simulink model "HANcoder_E407_TTA_Group2"  (R2018b)
settings: Solver=FixedStepDiscrete  StartTime=0.0  StopTime=1  FixedStep=0.01  RelTol=1e-3
PreLoadFcn:
  | librarySetup
  | eval([bdroot,'_startup']) %Calling [modelName]_startup.m
values from neighbouring files (symbols this model uses):
  BackUp_Role = 4    [HANcoder_E407_TTA_Group2_startup.m]
  basic_cycle_duration_bc0 = TM_Reset_Board   + COMP_duration    (= 550)    [HANcoder_E407_TTA_Group2_startup.m]    (also in HANcoder_E407_TTA_Template_startup.m = 212)
  basic_cycle_duration_bc1 = TM_Reset_Var_bc1 + COMP_duration    (= 610)    [HANcoder_E407_TTA_Group2_startup.m]    (also in HANcoder_E407_TTA_Template_startup.m = 212)
  board1_online = Simulink.Parameter    [HANcoder_E407_TTA_Group2_startup.m]
  board2_online = Simulink.Parameter    [HANcoder_E407_TTA_Group2_startup.m]
  board3_online = Simulink.Parameter    [HANcoder_E407_TTA_Group2_startup.m]
  board4_online = Simulink.Parameter    [HANcoder_E407_TTA_Group2_startup.m]
  comm_delay_estimation1 = round(comm_delay_measured1*hardware_granularity/frequency_IRQ)    [HANcoder_E407_TTA_Group2_startup.m]    (also in HANcoder_E407_TTA_Template_startup.m)
  comm_delay_estimation2 = round(comm_delay_measured2*hardware_granularity/frequency_IRQ)    [HANcoder_E407_TTA_Group2_startup.m]    (also in HANcoder_E407_TTA_Template_startup.m)
  COMM_Period = 50    [HANcoder_E407_TTA_Group2_startup.m]    (also in HANcoder_E407_TTA_Template_startup.m = 40)
  COMM_Phase1 = Simulink.Parameter    [HANcoder_E407_TTA_Group2_startup.m]    (also in HANcoder_E407_TTA_Template_startup.m)
  COMM_Phase2 = Simulink.Parameter    [HANcoder_E407_TTA_Group2_startup.m]    (also in HANcoder_E407_TTA_Template_startup.m)
  COMM_Phase_init1 = Simulink.Parameter    [HANcoder_E407_TTA_Group2_startup.m]    (also in HANcoder_E407_TTA_Template_startup.m)
  COMM_Phase_init2 = Simulink.Parameter    [HANcoder_E407_TTA_Group2_startup.m]    (also in HANcoder_E407_TTA_Template_startup.m)
  COMP_duration = 20    [HANcoder_E407_TTA_Group2_startup.m]    (also in HANcoder_E407_TTA_Template_startup.m = 4)
  Controller1_Board = 1    [HANcoder_E407_TTA_Group2_startup.m]    (also in HANcoder_E407_TTA_Template_startup.m)
  Controller2_Board = 2    [HANcoder_E407_TTA_Group2_startup.m]    (also in HANcoder_E407_TTA_Template_startup.m)
  Controller3_Board = 3    [HANcoder_E407_TTA_Group2_startup.m]    (also in HANcoder_E407_TTA_Template_startup.m)
  Controller4_Board = 4    [HANcoder_E407_TTA_Group2_startup.m]
  delta_a_set = Simulink.Parameter    [HANcoder_E407_TTA_Group2_startup.m]
  delta_f_set = Simulink.Parameter    [HANcoder_E407_TTA_Group2_startup.m]
  delta_max = 1    [HANcoder_E407_TTA_Group2_startup.m]
  delta_min = -1    [HANcoder_E407_TTA_Group2_startup.m]
  delta_precision = 6    [HANcoder_E407_TTA_Group2_startup.m]
  e_width = 0.1    [HANcoder_E407_TTA_Group2_startup.m]
  ErrorLog_ID = 31    [HANcoder_E407_TTA_Group2_startup.m]
  frequency_IRQ = 100    [HANcoder_E407_TTA_Group2_startup.m]    (also in HANcoder_E407_TTA_Template_startup.m)
  HANtuneOverride = Simulink.Parameter    [HANcoder_E407_TTA_Group2_startup.m]    (also in HANcoder_E407_TTA_Template_startup.m)
  hardware_granularity = 1000000    [HANcoder_E407_TTA_Group2_startup.m]    (also in HANcoder_E407_TTA_Template_startup.m)
  I_a = 2.25    [HANcoder_E407_TTA_Group2_startup.m]
  I_f = 2.25    [HANcoder_E407_TTA_Group2_startup.m]
  idle_time_init = basic_cycle_duration_bc0 + basic_cycle_duration_bc1    (= 1160)    [HANcoder_E407_TTA_Group2_startup.m]    (also in HANcoder_E407_TTA_Template_startup.m = 424)
  Input_Gen_Board = 5    [HANcoder_E407_TTA_Group2_startup.m]
  LA_Clock_Gr = 1    [HANcoder_E407_TTA_Group2_startup.m]    (also in HANcoder_E407_TTA_Template_startup.m)
  LA_COMM_dly = 1    [HANcoder_E407_TTA_Group2_startup.m]    (also in HANcoder_E407_TTA_Template_startup.m)
  LA_COMM_Err = 1    [HANcoder_E407_TTA_Group2_startup.m]    (also in HANcoder_E407_TTA_Template_startup.m)
  LA_E_Desync = 1    [HANcoder_E407_TTA_Group2_startup.m]    (also in HANcoder_E407_TTA_Template_startup.m)
  LA_MEX_Flag = 1    [HANcoder_E407_TTA_Group2_startup.m]    (also in HANcoder_E407_TTA_Template_startup.m)
  LA_Task_Act = 1    [HANcoder_E407_TTA_Group2_startup.m]    (also in HANcoder_E407_TTA_Template_startup.m)
  m_v = 100.0    (= 100)    [HANcoder_E407_TTA_Group2_startup.m]
  Master_Role = 1    [HANcoder_E407_TTA_Group2_startup.m]    (also in HANcoder_E407_TTA_Template_startup.m)
  matrix_cycle_duration = basic_cycle_duration_bc0 + basic_cycle_duration_bc1    (= 1160)    [HANcoder_E407_TTA_Group2_startup.m]    (also in HANcoder_E407_TTA_Template_startup.m = 424)
  matrix_rows = 2    [HANcoder_E407_TTA_Group2_startup.m]    (also in HANcoder_E407_TTA_Template_startup.m)
  max_desync = 15    [HANcoder_E407_TTA_Group2_startup.m]    (also in HANcoder_E407_TTA_Template_startup.m)
  max_num_msgs_CAN1 = 2^Tx_bit_number-1    (= 7)    [HANcoder_E407_TTA_Group2_startup.m]    (also in HANcoder_E407_TTA_Template_startup.m)
  max_num_msgs_CAN2 = max_num_msgs_CAN1    (= 7)    [HANcoder_E407_TTA_Group2_startup.m]    (also in HANcoder_E407_TTA_Template_startup.m)
  min_desync = (-1)*max_desync    (= -15)    [HANcoder_E407_TTA_Group2_startup.m]    (also in HANcoder_E407_TTA_Template_startup.m)
  OutControl1_ID = 23    [HANcoder_E407_TTA_Group2_startup.m]    (also in HANcoder_E407_TTA_Template_startup.m)
  OutControl2_ID = 24    [HANcoder_E407_TTA_Group2_startup.m]    (also in HANcoder_E407_TTA_Template_startup.m)
  OutEmulator_ID = 25    [HANcoder_E407_TTA_Group2_startup.m]    (also in HANcoder_E407_TTA_Template_startup.m)
  R_al = 0.10    (= 0.1)    [HANcoder_E407_TTA_Group2_startup.m]
  R_ar = 0.10    (= 0.1)    [HANcoder_E407_TTA_Group2_startup.m]
  R_fl = 0.10    (= 0.1)    [HANcoder_E407_TTA_Group2_startup.m]
  R_fr = 0.10    (= 0.1)    [HANcoder_E407_TTA_Group2_startup.m]
  script_run = Simulink.Parameter    [HANcoder_E407_TTA_Group2_startup.m]    (also in HANcoder_E407_TTA_Template_startup.m)
  SensorValues_ID = 22    [HANcoder_E407_TTA_Group2_startup.m]    (also in HANcoder_E407_TTA_Template_startup.m)
  SetValues_ID = 21    [HANcoder_E407_TTA_Group2_startup.m]    (also in HANcoder_E407_TTA_Template_startup.m)
  Slave_Role = 3    [HANcoder_E407_TTA_Group2_startup.m]    (also in HANcoder_E407_TTA_Template_startup.m = 2)
  speed_k_d = Simulink.Parameter    [HANcoder_E407_TTA_Group2_startup.m]
  speed_k_i = Simulink.Parameter    [HANcoder_E407_TTA_Group2_startup.m]
  speed_k_p = Simulink.Parameter    [HANcoder_E407_TTA_Group2_startup.m]
  speed_max = 10    [HANcoder_E407_TTA_Group2_startup.m]
  speed_min = -10    [HANcoder_E407_TTA_Group2_startup.m]
  speed_precision = 3    [HANcoder_E407_TTA_Group2_startup.m]
  Sync_ID = 1    [HANcoder_E407_TTA_Group2_startup.m]    (also in HANcoder_E407_TTA_Template_startup.m)
  tau_max = 5    [HANcoder_E407_TTA_Group2_startup.m]
  tau_min = -5    [HANcoder_E407_TTA_Group2_startup.m]
  tau_range = abs(tau_max) + abs(tau_min)    [HANcoder_E407_TTA_Group2_startup.m]
  theta_max = (speed_max/R_fr)*matrix_cycle_duration*frequency_IRQ/hardware_granularity    (= 11.6)    [HANcoder_E407_TTA_Group2_startup.m]
  theta_min = (-1)*theta_max    (= -11.6)    [HANcoder_E407_TTA_Group2_startup.m]
  theta_precision = 7-(fix(log2(theta_max))+1)    [HANcoder_E407_TTA_Group2_startup.m]
  Tl_a = 0.6    [HANcoder_E407_TTA_Group2_startup.m]
  Tl_f = 0.6    [HANcoder_E407_TTA_Group2_startup.m]
  TM_bc0_1 = basic_cycle_start    (= 0)    [HANcoder_E407_TTA_Group2_startup.m]
  TM_bc0_10 = TM_bc0_9 + COMP_duration    (= 270)    [HANcoder_E407_TTA_Group2_startup.m]
  TM_bc0_11 = TM_bc0_10 + COMP_duration    (= 290)    [HANcoder_E407_TTA_Group2_startup.m]
  TM_bc0_12 = TM_bc0_11  + COMM_duration    (= 340)    [HANcoder_E407_TTA_Group2_startup.m]
  TM_bc0_13 = TM_bc0_12 + COMP_duration    (= 360)    [HANcoder_E407_TTA_Group2_startup.m]
  TM_bc0_14 = TM_bc0_13 + COMP_duration    (= 380)    [HANcoder_E407_TTA_Group2_startup.m]
  TM_bc0_15 = TM_bc0_14  + COMM_duration    (= 430)    [HANcoder_E407_TTA_Group2_startup.m]
  TM_bc0_16 = TM_bc0_15 + COMP_duration    (= 450)    [HANcoder_E407_TTA_Group2_startup.m]
  TM_bc0_17 = TM_bc0_16 + COMP_duration    (= 470)    [HANcoder_E407_TTA_Group2_startup.m]
  TM_bc0_18 = TM_bc0_17 + COMP_duration    (= 490)    [HANcoder_E407_TTA_Group2_startup.m]
  TM_bc0_2 = TM_bc0_1   + COMM_duration    (= 50)    [HANcoder_E407_TTA_Group2_startup.m]
  TM_bc0_3 = TM_bc0_2  + COMP_duration    (= 70)    [HANcoder_E407_TTA_Group2_startup.m]
  TM_bc0_3_2 = TM_bc0_3   + 2    (= 72)    [HANcoder_E407_TTA_Group2_startup.m]
  TM_bc0_4 = TM_bc0_3   + COMP_duration    (= 90)    [HANcoder_E407_TTA_Group2_startup.m]
  TM_bc0_4_2 = TM_bc0_4    + 2    (= 92)    [HANcoder_E407_TTA_Group2_startup.m]
  TM_bc0_5 = TM_bc0_4    + COMP_duration    (= 110)    [HANcoder_E407_TTA_Group2_startup.m]
  TM_bc0_6 = TM_bc0_5  + COMM_duration    (= 160)    [HANcoder_E407_TTA_Group2_startup.m]
  TM_bc0_7 = TM_bc0_6 + COMP_duration    (= 180)    [HANcoder_E407_TTA_Group2_startup.m]
  TM_bc0_8 = TM_bc0_7 + COMP_duration    (= 200)    [HANcoder_E407_TTA_Group2_startup.m]
  TM_bc0_9 = TM_bc0_8  + COMM_duration    (= 250)    [HANcoder_E407_TTA_Group2_startup.m]
  TM_bc0_9_2 = TM_bc0_9 + 2    (= 252)    [HANcoder_E407_TTA_Group2_startup.m]
  TM_bc1_18 = TM_Check_Output_Emulator + COMP_duration    (= 520)    [HANcoder_E407_TTA_Group2_startup.m]
  TM_bc1_19 = TM_bc1_18 + COMM_duration    (= 570)    [HANcoder_E407_TTA_Group2_startup.m]
  TM_bc1_19_2 = TM_bc1_19 + 2    (= 572)    [HANcoder_E407_TTA_Group2_startup.m]
  TM_Check_Output_Control1 = TM_COMM_Output_Control1 + COMP_duration    (= 340)    [HANcoder_E407_TTA_Group2_startup.m]
  TM_Check_Output_Control2 = TM_COMM_Output_Control2 + COMM_duration    (= 410)    [HANcoder_E407_TTA_Group2_startup.m]
  TM_Check_Output_Emulator = TM_COMM_Output_Emulator + COMM_duration    (= 500)    [HANcoder_E407_TTA_Group2_startup.m]
  TM_Check_Output_Emulator_2 = TM_Check_Output_Emulator + 2    (= 502)    [HANcoder_E407_TTA_Group2_startup.m]
  TM_Check_Sensor_Values = TM_COMM_Sensor_Values + COMM_duration    (= 210)    [HANcoder_E407_TTA_Group2_startup.m]
  TM_Check_Sensor_Values_2 = TM_Check_Sensor_Values + 2    (= 212)    [HANcoder_E407_TTA_Group2_startup.m]
  TM_Check_Set_Values = TM_COMM_Set_Values + COMM_duration    (= 140)    [HANcoder_E407_TTA_Group2_startup.m]
  TM_Check_Set_Values_2 = TM_Check_Set_Values + 2    (= 142)    [HANcoder_E407_TTA_Group2_startup.m]
  TM_COMM_Output_Control1 = TM_Velocity + COMM_duration    (= 320)    [HANcoder_E407_TTA_Group2_startup.m]
  TM_COMM_Output_Control2 = TM_Check_Output_Control1 + COMP_duration    (= 360)    [HANcoder_E407_TTA_Group2_startup.m]
  TM_COMM_Output_Emulator = TM_TMR + COMP_duration    (= 450)    [HANcoder_E407_TTA_Group2_startup.m]
  TM_COMM_Sensor_Values = TM_Check_Set_Values + COMP_duration    (= 160)    [HANcoder_E407_TTA_Group2_startup.m]
  TM_COMM_Set_Values = TM_bc0_3 + COMP_duration    (= 90)    [HANcoder_E407_TTA_Group2_startup.m]
  TM_COMM_Sync = basic_cycle_start    (= 0)    [HANcoder_E407_TTA_Group2_startup.m]    (also in HANcoder_E407_TTA_Template_startup.m)
  TM_Data_bc0 = TM_COMM_Sync    (= 0)    [HANcoder_E407_TTA_Group2_startup.m]    (also in HANcoder_E407_TTA_Template_startup.m)
  TM_Data_bc1 = TM_Data_bc0(1:4)    [HANcoder_E407_TTA_Group2_startup.m]    (also in HANcoder_E407_TTA_Template_startup.m)
  TM_Reset_Board = TM_Reset_Var   + COMP_duration    (= 530)    [HANcoder_E407_TTA_Group2_startup.m]    (also in HANcoder_E407_TTA_Template_startup.m = 208)
  TM_Reset_Var = TM_bc0_18  + COMP_duration    (= 510)    [HANcoder_E407_TTA_Group2_startup.m]    (also in HANcoder_E407_TTA_Template_startup.m = 204)
  TM_Reset_Var_bc1 = TM_bc1_19 + COMP_duration    (= 590)    [HANcoder_E407_TTA_Group2_startup.m]    (also in HANcoder_E407_TTA_Template_startup.m = 200)
  TM_Reset_Var_bc1_2 = TM_Reset_Var_bc1 + 2    (= 592)    [HANcoder_E407_TTA_Group2_startup.m]    (also in HANcoder_E407_TTA_Template_startup.m = 202)
  TM_Steer = TM_Check_Sensor_Values + COMP_duration    (= 230)    [HANcoder_E407_TTA_Group2_startup.m]
  TM_TMR = TM_Check_Output_Control2 + COMP_duration    (= 430)    [HANcoder_E407_TTA_Group2_startup.m]
  TM_TMR_2 = TM_TMR + 1    (= 431)    [HANcoder_E407_TTA_Group2_startup.m]
  ... (+19 more)
undefined symbols (not defined in the file or in its folder): A0, A1, A2, A3, A4, CON2, CON4, D10, D12, D13, D8, D9
libraries: hdlsllib x340, HANcoder_STM32_Target x28, simulink x5, simulink_extras x1
(part 27 of 36)

== system HANcoder_E407_TTA_Group2/HANcoder STM32 Target - E407-STM32 algorithm/TTA CAN System/TTA System/Matrix Cycle Manager/Vehicle Emulator Matrix Cycle/vehicle emulator basic cycle 1/COMM Task - Sensor_Values/Transmission subtasks/Check msg transmission CAN2 ==
  note: In the next tick, a message will be
      | sent through CAN2
  note: A message should be sent during
      | this tick through CAN2
  note: The TX buffers are updated one tick
      | before the message is sent
  Local Time : Inport
  Time Mark : Inport  Port=2
  Tx_ID : Inport  Port=3
  Value Domain Msg : Inport  Port=4
  Enable : EnablePort
  Constant : Constant  Value=COMM_Phase_init2
  Constant11 : Constant  Value=0
  Constant22 : Constant
  Constant24 : Constant  Value=COMM_Phase2
  Constant27 : Constant  Value=COMM_Phase2
  Constant8 : Constant  Value=0
  Equal4 : RelationalOperator  Operator===  OutDataTypeStr=boolean  RndMeth=Simplest
  Equal7 : RelationalOperator  Operator===  OutDataTypeStr=boolean  RndMeth=Simplest
  Minus : Sum  Inputs=++-
  Minus1 : Sum  Inputs=+-
  Minus2 : Sum
  Mod : Math  Operator=mod  SaturateOnIntegerOverflow=on
  Mod1 : Math  Operator=mod  SaturateOnIntegerOverflow=on
  TX buffer update CAN2 : Subsystem  Priority=20
  Send CAN2 : Outport  OutputWhenDisabled=reset  InitialOutput=0
  wires:
  Constant8/1 -> Equal4/2
  Equal7/1 -> Send CAN2/1
  Constant11/1 -> Equal7/2
  Minus1/1 -> Mod1/1
  Mod/1 -> Equal4/1
  Constant24/1 -> Mod/2
  Value Domain Msg/1 -> TX buffer update CAN2/2(Msg_Value_Data)
  Minus/1 -> Mod/1
  Constant27/1 -> Mod1/2
  Mod1/1 -> Equal7/1
  Tx_ID/1 -> TX buffer update CAN2/1(Tx_ID)
  Local Time/1 -> Minus/1, Minus1/1
  Constant22/1 -> Minus/2
  Equal4/1 -> TX buffer update CAN2/Enable
  Constant/1 -> Minus2/2
  Time Mark/1 -> Minus2/1
  Minus2/1 -> Minus1/2, Minus/3

== system HANcoder_E407_TTA_Group2/HANcoder STM32 Target - E407-STM32 algorithm/TTA CAN System/TTA System/Matrix Cycle Manager/Vehicle Emulator Matrix Cycle/vehicle emulator basic cycle 1/COMM Task - Sensor_Values/Transmission subtasks/Msg_Value_Data_Encoded ==
  note: Value domain message encoding
      | <Warning!> The first buffer (from the top) is not used in transmission!
  Enable : EnablePort
  Bus Creator : BusCreator  Inputs=8  OutDataTypeStr=Bus: msg_buffer_type
  Constant : Constant  Value=0  OutDataTypeStr=uint8
  Constant{1,7,10,13} (4 alike) : Constant  Value=theta_precision
  Constant{5,8,11,14} (4 alike) : Constant  Value=theta_max
  Constant{6,9,12,15} (4 alike) : Constant  Value=theta_min
  Data Store Read1 : DataStoreRead  DataStoreName=theta_fl_incr
  Data Store Read2 : DataStoreRead  DataStoreName=theta_ar_incr
  Data Store Read3 : DataStoreRead  DataStoreName=theta_al_incr
  Data Store Read5 : DataStoreRead  DataStoreName=theta_fr_incr
  float2uint1 : Subsystem
  float2uint2 : Subsystem
  float2uint3 : Subsystem
  float2uint4 : Subsystem
  Value_domain_msg : Outport
  wires:
  Bus Creator/1 -> Value_domain_msg/1
  Constant1/1 -> float2uint2/1(precision)
  Constant/1 -> Bus Creator/1, Bus Creator/6, Bus Creator/7, Bus Creator/8
  float2uint2/1(coded) -> Bus Creator/2
  Constant5/1 -> float2uint2/3(magnitude_max)
  Constant6/1 -> float2uint2/4(magnitude_min)
  Constant9/1 -> float2uint1/4(magnitude_min)
  Constant8/1 -> float2uint1/3(magnitude_max)
  Constant7/1 -> float2uint1/1(precision)
  float2uint1/1(coded) -> Bus Creator/3
  Constant10/1 -> float2uint3/1(precision)
  Constant11/1 -> float2uint3/3(magnitude_max)
  Constant12/1 -> float2uint3/4(magnitude_min)
  float2uint3/1(coded) -> Bus Creator/4
  Constant15/1 -> float2uint4/4(magnitude_min)
  Constant14/1 -> float2uint4/3(magnitude_max)
  Constant13/1 -> float2uint4/1(precision)
  float2uint4/1(coded) -> Bus Creator/5
  Data Store Read5/1 -> float2uint2/2(magnitude)
  Data Store Read1/1 -> float2uint1/2(magnitude)
  Data Store Read2/1 -> float2uint3/2(magnitude)
  Data Store Read3/1 -> float2uint4/2(magnitude)

== system HANcoder_E407_TTA_Group2/HANcoder STM32 Target - E407-STM32 algorithm/TTA CAN System/TTA System/Matrix Cycle Manager/Vehicle Emulator Matrix Cycle/vehicle emulator basic cycle 1/COMM Task - Sync bc 1/Reception substasks/RX buffers update ==
  note: Reset RX Buffer Flag
  note: Reception ID
      |    Sync Msg: 1
      |    Vote Node 1: 11
      |    Vote Node 2: 12
      |    Vote Node 3: 13
  note: Wait until new message
      | arrives
  note: Reset RX Buffer Flag
  note: Reception ID
      |    Sync Msg: 1
      |    Vote Node 1: 11
      |    Vote Node 2: 12
      |    Vote Node 3: 13
  note: Wait until new message
      | arrives
  note: Reset Rx buffers
  note: Reception end - Set RxID and Reset CAN buffer flags
  note: CAN1
  note: CAN2
  Rx_ID : Inport
  Enable : EnablePort
  Cast13 : DataTypeConversion  OutDataTypeStr=uint32
  Cast14 : DataTypeConversion  OutDataTypeStr=boolean
  Cast15 : DataTypeConversion  OutDataTypeStr=uint8
  Cast3 : DataTypeConversion  OutDataTypeStr=uint32
  Cast5 : DataTypeConversion  OutDataTypeStr=boolean
  Cast6 : DataTypeConversion  OutDataTypeStr=uint8
  Data Store Write : DataStoreWrite  DataStoreName=Msg_Rx
  Data Store Write11 : DataStoreWrite  DataStoreName=RxID_CAN2
  Data Store Write12 : DataStoreWrite  DataStoreName=Rx_State_CAN2
  Data Store Write2 : DataStoreWrite  DataStoreName=New_Msg_Ready_CAN1
  Data Store Write3 : DataStoreWrite  DataStoreName=new_msg_Rx
  Data Store Write6 : DataStoreWrite  DataStoreName=RxID_CAN1
  Data Store Write7 : DataStoreWrite  DataStoreName=Rx_State_CAN1
  Data Store Write9 : DataStoreWrite  DataStoreName=New_Msg_Ready_CAN2
  RESET1 : Constant  Value=0
  RESET2 : Constant  Value=0
  RESET_CAN1_new_buffer : Constant  Value=0
  RESET_CAN2_new_buffer : Constant  Value=0
  RESET_Msg_Rx : Constant  Value=0  OutDataTypeStr=Bus: msg_buffer_type
  RESET_new_msg_Rx : Constant  Value=0  OutDataTypeStr=boolean
  wires:
  Cast13/1 -> Data Store Write11/1
  Rx_ID/1 -> Cast3/1, Cast13/1
  RESET2/1 -> Cast14/1
  Cast14/1 -> Data Store Write9/1
  RESET_CAN2_new_buffer/1 -> Cast15/1
  Cast15/1 -> Data Store Write12/1
  Cast6/1 -> Data Store Write7/1
  RESET_CAN1_new_buffer/1 -> Cast6/1
  RESET_new_msg_Rx/1 -> Data Store Write3/1
  RESET_Msg_Rx/1 -> Data Store Write/1
  Cast5/1 -> Data Store Write2/1
  RESET1/1 -> Cast5/1
  Cast3/1 -> Data Store Write6/1

== system HANcoder_E407_TTA_Group2/HANcoder STM32 Target - E407-STM32 algorithm/TTA CAN System/TTA System/Matrix Cycle Manager/Vehicle Emulator Matrix Cycle/vehicle emulator basic cycle 1/COMM Task - Sync bc 1/Transmission subtasks/Check msg transmission CAN1 ==
  note: The TX buffers are updated one tick
      | before the message is sent
  note: A message should be sent during
      | this tick through CAN1
  note: In the next tick, a message will be
      | sent through CAN1
  Local Time : Inport
  Time Mark : Inport  Port=2
  Tx_ID : Inport  Port=3
  Value Domain Msg : Inport  Port=4
  Enable : EnablePort
  Constant : Constant  Value=COMM_Phase_init1
  Constant11 : Constant  Value=0
  Constant22 : Constant
  Constant24 : Constant  Value=COMM_Phase1
  Constant27 : Constant  Value=COMM_Phase1
  Constant8 : Constant  Value=0
  Equal4 : RelationalOperator  Operator===  OutDataTypeStr=boolean  RndMeth=Simplest
  Equal7 : RelationalOperator  Operator===  OutDataTypeStr=boolean  RndMeth=Simplest
  Minus : Sum  Inputs=++-
  Minus1 : Sum  Inputs=+-
  Minus2 : Sum
  Mod : Math  Operator=mod  SaturateOnIntegerOverflow=on
  Mod1 : Math  Operator=mod  SaturateOnIntegerOverflow=on
  TX buffer update CAN1 : Subsystem  Priority=20
  Send CAN1 : Outport  OutputWhenDisabled=reset  InitialOutput=0
  wires:
  Equal4/1 -> TX buffer update CAN1/Enable
  Constant22/1 -> Minus/2
  Local Time/1 -> Minus1/1, Minus/1
  Tx_ID/1 -> TX buffer update CAN1/1(Tx_ID)
  Mod1/1 -> Equal7/1
  Constant27/1 -> Mod1/2
  Minus/1 -> Mod/1
  Value Domain Msg/1 -> TX buffer update CAN1/2(Msg_Value_Data)
  Constant24/1 -> Mod/2
  Mod/1 -> Equal4/1
  Minus1/1 -> Mod1/1
  Constant11/1 -> Equal7/2
  Equal7/1 -> Send CAN1/1
  Constant8/1 -> Equal4/2
  Constant/1 -> Minus2/2
  Minus2/1 -> Minus1/2, Minus/3
  Time Mark/1 -> Minus2/1

== system HANcoder_E407_TTA_Group2/HANcoder STM32 Target - E407-STM32 algorithm/TTA CAN System/TTA System/Matrix Cycle Manager/Vehicle Emulator Matrix Cycle/vehicle emulator basic cycle 1/COMM Task - Sync bc 1/Transmission subtasks/Check msg transmission CAN2 ==
  note: In the next tick, a message will be
      | sent through CAN2
  note: A message should be sent during
      | this tick through CAN2
  note: The TX buffers are updated one tick
      | before the message is sent
  Local Time : Inport
  Time Mark : Inport  Port=2
  Tx_ID : Inport  Port=3
  Value Domain Msg : Inport  Port=4
  Enable : EnablePort
  Constant : Constant  Value=COMM_Phase_init2
  Constant11 : Constant  Value=0
  Constant22 : Constant
  Constant24 : Constant  Value=COMM_Phase2
  Constant27 : Constant  Value=COMM_Phase2
  Constant8 : Constant  Value=0
  Equal4 : RelationalOperator  Operator===  OutDataTypeStr=boolean  RndMeth=Simplest
  Equal7 : RelationalOperator  Operator===  OutDataTypeStr=boolean  RndMeth=Simplest
  Minus : Sum  Inputs=++-
  Minus1 : Sum  Inputs=+-
  Minus2 : Sum
  Mod : Math  Operator=mod  SaturateOnIntegerOverflow=on
  Mod1 : Math  Operator=mod  SaturateOnIntegerOverflow=on
  TX buffer update CAN2 : Subsystem  Priority=20
  Send CAN2 : Outport  OutputWhenDisabled=reset  InitialOutput=0
  wires:
  Constant8/1 -> Equal4/2
  Equal7/1 -> Send CAN2/1
  Constant11/1 -> Equal7/2
  Minus1/1 -> Mod1/1
  Mod/1 -> Equal4/1
  Constant24/1 -> Mod/2
  Value Domain Msg/1 -> TX buffer update CAN2/2(Msg_Value_Data)
  Minus/1 -> Mod/1
  Constant27/1 -> Mod1/2
  Mod1/1 -> Equal7/1
  Tx_ID/1 -> TX buffer update CAN2/1(Tx_ID)
  Local Time/1 -> Minus/1, Minus1/1
  Constant22/1 -> Minus/2
  Equal4/1 -> TX buffer update CAN2/Enable
  Constant/1 -> Minus2/2
  Time Mark/1 -> Minus2/1
  Minus2/1 -> Minus1/2, Minus/3

== system HANcoder_E407_TTA_Group2/HANcoder STM32 Target - E407-STM32 algorithm/TTA CAN System/TTA System/Matrix Cycle Manager/Vehicle Emulator Matrix Cycle/vehicle emulator basic cycle 1/COMM Task - Sync bc 1/Transmission subtasks/Msg_Value_Data_Encoded ==
  note: Value domain message encoding
      | <Warning!> The first buffer (from the top) is not used in transmission!
  Enable : EnablePort
  Bus Creator : BusCreator  Inputs=8  OutDataTypeStr=Bus: msg_buffer_type
  Constant : Constant  Value=0  OutDataTypeStr=uint8
  Value_domain_msg : Outport
  wires:
  Bus Creator/1 -> Value_domain_msg/1
  Constant/1 -> Bus Creator/1, Bus Creator/2, Bus Creator/3, Bus Creator/4, Bus Creator/5, Bus Creator/8, Bus Creator/7, Bus Creator/6

== system HANcoder_E407_TTA_Group2/HANcoder STM32 Target - E407-STM32 algorithm/TTA CAN System/TTA System/Matrix Cycle Manager/Vehicle Emulator Matrix Cycle/vehicle emulator basic cycle 1/COMP Task - Rx Output Emulator Check/Process_Messages/Demux message CAN1 and check coherence ==
  CAN1_Rx_msg : Inport  OutDataTypeStr=Bus: msg_buffer_type
  expected_board_id : Inport  Port=2
  Enable : EnablePort
  Bus Creator : BusCreator  Inputs=8  OutDataTypeStr=Bus: msg_buffer_type
  Bus Selector : BusSelector  OutputSignals=Buffer_1,Buffer_2,Buffer_3,Buffer_4,Buffer_5,Buffer_6,Buffer_7,Buffer_8
  Constant : Constant  Value=0  OutDataTypeStr=uint8
  Equal : RelationalOperator  Operator===  OutDataTypeStr=boolean  RndMeth=Simplest
  Subsystem : Subsystem
  Terminator : Terminator
  msg_count>2_DEBUG : Subsystem
  CAN1_msg : Outport  OutDataTypeStr=Bus: msg_buffer_type
  Msg_Count_CAN1 : Outport  Port=2
  CAN1_msg_coherent : Outport  Port=3  OutputWhenDisabled=reset  InitialOutput=0
  wires:
  Bus Selector/2 -> Bus Creator/2  "<Buffer_2>"
  Bus Selector/3 -> Bus Creator/3  "<Buffer_3>"
  CAN1_Rx_msg/1 -> Bus Selector/1
  Equal/1 -> CAN1_msg_coherent/1
  expected_board_id/1 -> Equal/2
  Bus Selector/6 -> Bus Creator/6  "<Buffer_6>"
  Bus Selector/5 -> Bus Creator/5  "<Buffer_5>"
  Bus Selector/7 -> Bus Creator/7  "<Buffer_7>"
  Bus Selector/8 -> Bus Creator/8  "<Buffer_8>"
  Bus Selector/4 -> Bus Creator/4  "<Buffer_4>"
  Subsystem/3(board_id) -> Equal/1
  Bus Selector/1 -> Subsystem/1(Msg_Temporal_Data)  "<Buffer_1>"
  Subsystem/2(msg_count) -> msg_count>2_DEBUG/1(msg_c), Msg_Count_CAN1/1
  Bus Creator/1 -> CAN1_msg/1
  Constant/1 -> Bus Creator/1
  Subsystem/1(basic_cycle) -> Terminator/1

== system HANcoder_E407_TTA_Group2/HANcoder STM32 Target - E407-STM32 algorithm/TTA CAN System/TTA System/Matrix Cycle Manager/Vehicle Emulator Matrix Cycle/vehicle emulator basic cycle 1/COMP Task - Rx Output Emulator Check/Process_Messages/Demux message CAN1 and check coherence1 ==
  CAN2_Rx_msg : Inport  OutDataTypeStr=Bus: msg_buffer_type
  expected_board_id : Inport  Port=2
  Enable : EnablePort
  Bus Creator : BusCreator  Inputs=8  OutDataTypeStr=Bus: msg_buffer_type
  Bus Selector : BusSelector  OutputSignals=Buffer_1,Buffer_2,Buffer_3,Buffer_4,Buffer_5,Buffer_6,Buffer_7,Buffer_8
  Constant : Constant  Value=0  OutDataTypeStr=uint8
  Equal : RelationalOperator  Operator===  OutDataTypeStr=boolean  RndMeth=Simplest
  Subsystem : Subsystem
  Terminator : Terminator
  msg_count>2_DEBUG : Subsystem
  CAN2_msg_coherent : Outport  OutputWhenDisabled=reset  InitialOutput=0
  Msg_Count_CAN2 : Outport  Port=2
  CAN2_msg : Outport  Port=3  OutDataTypeStr=Bus: msg_buffer_type
  wires:
  Bus Selector/2 -> Bus Creator/2  "<Buffer_2>"
  Bus Selector/3 -> Bus Creator/3  "<Buffer_3>"
  CAN2_Rx_msg/1 -> Bus Selector/1
  Equal/1 -> CAN2_msg_coherent/1
  expected_board_id/1 -> Equal/2
  Bus Selector/6 -> Bus Creator/6  "<Buffer_6>"
  Bus Selector/5 -> Bus Creator/5  "<Buffer_5>"
  Bus Selector/7 -> Bus Creator/7  "<Buffer_7>"
  Bus Selector/8 -> Bus Creator/8  "<Buffer_8>"
  Bus Selector/4 -> Bus Creator/4  "<Buffer_4>"
  Subsystem/3(board_id) -> Equal/1
  Bus Selector/1 -> Subsystem/1(Msg_Temporal_Data)  "<Buffer_1>"
  Subsystem/2(msg_count) -> msg_count>2_DEBUG/1(msg_c), Msg_Count_CAN2/1
  Bus Creator/1 -> CAN2_msg/1
  Constant/1 -> Bus Creator/1
  Subsystem/1(basic_cycle) -> Terminator/1

== system HANcoder_E407_TTA_Group2/HANcoder STM32 Target - E407-STM32 algorithm/TTA CAN System/TTA System/Matrix Cycle Manager/Vehicle Emulator Matrix Cycle/vehicle emulator basic cycle 1/COMP Task - Rx Output Emulator Check/Update Msg buffer/Sensor Values Rx Update ==
  note: If we miss any msg, with current version we
      | suppose vehicle emulator remains in the same
      | state until new msg is received.
  note: Reinitialize variables
  note: Ticks to seconds conversion
  note: Matrix cycles since last input value
  note: For derivatives and integrals it is important to keep
      | track of how much time has passed since the last
      | time we received a controller value.
  msg_rx : Inport
  Enable : EnablePort
  Bus Selector : BusSelector  OutputSignals=Buffer_2,Buffer_3,Buffer_4,Buffer_5
  Constant : Constant  Value=matrix_cycle_duration
  Constant{1..4} (4 alike) : Constant  Value=torque_precision
  Constant5 : Constant
  Constant6 : Constant  Value=0  OutDataTypeStr=boolean
  Constant7 : Constant
  Data Store Read1 : DataStoreRead  DataStoreName=mc_counter
  Data Store Write : DataStoreWrite  DataStoreName=torque_fr
  Data Store Write1 : DataStoreWrite  DataStoreName=torque_fl
  Data Store Write2 : DataStoreWrite  DataStoreName=torque_ar
  Data Store Write3 : DataStoreWrite  DataStoreName=torque_al
  Data Store Write4 : DataStoreWrite  Priority=1  DataStoreName=rx_data_incr_time
  Data Store Write5 : DataStoreWrite  Priority=2  DataStoreName=mc_counter
  Data Store Write6 : DataStoreWrite  DataStoreName=controller_msg_missed
  Gain : Gain  Gain=frequency_IRQ/hardware_granularity
  Multiply : Product
  Terminator : Terminator
  uint8_2float : Subsystem
  uint8_2float1 : Subsystem
  uint8_2float2 : Subsystem
  uint8_2float3 : Subsystem
  wires:
  msg_rx/1 -> Bus Selector/1
  Bus Selector/3 -> uint8_2float2/2(value)  "<Buffer_4>"
  Bus Selector/2 -> uint8_2float1/2(value)  "<Buffer_3>"
  Bus Selector/1 -> uint8_2float/2(value)  "<Buffer_2>"
  Bus Selector/4 -> uint8_2float3/2(value)  "<Buffer_5>"
  Constant4/1 -> uint8_2float/1(precision)
  Constant1/1 -> uint8_2float1/1(precision)
  Constant2/1 -> uint8_2float2/1(precision)
  Constant3/1 -> uint8_2float3/1(precision)
  uint8_2float3/1(decoded) -> Data Store Write3/1
  uint8_2float2/1(decoded) -> Data Store Write2/1
  uint8_2float1/1(decoded) -> Data Store Write1/1
  uint8_2float/1(decoded) -> Data Store Write/1
  Constant5/1 -> Data Store Write5/1
  Gain/1 -> Multiply/1
  Constant7/1 -> Multiply/2
  Multiply/1 -> Data Store Write4/1
  Constant/1 -> Gain/1
  Constant6/1 -> Data Store Write6/1
  Data Store Read1/1 -> Terminator/1

== system HANcoder_E407_TTA_Group2/HANcoder STM32 Target - E407-STM32 algorithm/TTA CAN System/TTA System/Matrix Cycle Manager/Vehicle Emulator Matrix Cycle/vehicle emulator basic cycle 1/COMP Task - Rx Output Emulator Check/Update Msg buffer/Sensor Values not Rx Update ==
  note: If no inputs received, no calculations are done.
      | Next time controller values are received
      | it is important to keep track of how much time
      | has passed for derivatives and integrals.
  Enable : EnablePort
  Constant1 : Constant
  Constant2 : Constant  OutDataTypeStr=boolean
  Data Store Read : DataStoreRead  DataStoreName=mc_counter
  Data Store Write : DataStoreWrite  DataStoreName=controller_msg_missed
  Data Store Write1 : DataStoreWrite  DataStoreName=mc_counter
  Minus : Sum
  wires:
  Minus/1 -> Data Store Write1/1
  Constant1/1 -> Minus/2
  Data Store Read/1 -> Minus/1
  Constant2/1 -> Data Store Write/1

== system HANcoder_E407_TTA_Group2/HANcoder STM32 Target - E407-STM32 algorithm/TTA CAN System/TTA System/Matrix Cycle Manager/Vehicle Emulator Matrix Cycle/vehicle emulator basic cycle 1/COMP Task - Sync bc1 check/Process_Messages/Demux message CAN1 and check coherence ==
  CAN1_Rx_msg : Inport  OutDataTypeStr=Bus: msg_buffer_type
  expected_basic_cycle : Inport  Port=2
  Enable : EnablePort
  Bus Creator : BusCreator  Inputs=8  OutDataTypeStr=Bus: msg_buffer_type
  Bus Selector : BusSelector  OutputSignals=Buffer_1,Buffer_2,Buffer_3,Buffer_4,Buffer_5,Buffer_6,Buffer_7,Buffer_8
  Constant : Constant  Value=0  OutDataTypeStr=uint8
  Equal1 : RelationalOperator  Operator===  OutDataTypeStr=boolean  RndMeth=Simplest
  Subsystem : Subsystem
  Terminator : Terminator
  msg_count>2_DEBUG : Subsystem
  CAN1_msg : Outport  OutDataTypeStr=Bus: msg_buffer_type
  Msg_Count_CAN1 : Outport  Port=2
  CAN1_msg_coherent : Outport  Port=3  OutputWhenDisabled=reset  InitialOutput=0
  wires:
  Bus Selector/2 -> Bus Creator/2  "<Buffer_2>"
  Bus Selector/3 -> Bus Creator/3  "<Buffer_3>"
  CAN1_Rx_msg/1 -> Bus Selector/1
  Equal1/1 -> CAN1_msg_coherent/1
  expected_basic_cycle/1 -> Equal1/2
  Bus Selector/6 -> Bus Creator/6  "<Buffer_6>"
  Bus Selector/5 -> Bus Creator/5  "<Buffer_5>"
  Bus Selector/7 -> Bus Creator/7  "<Buffer_7>"
  Bus Selector/8 -> Bus Creator/8  "<Buffer_8>"
  Bus Selector/4 -> Bus Creator/4  "<Buffer_4>"
  Bus Selector/1 -> Subsystem/1(Msg_Temporal_Data)  "<Buffer_1>"
  Subsystem/1(basic_cycle) -> Equal1/1
  Subsystem/2(msg_count) -> msg_count>2_DEBUG/1(msg_c), Msg_Count_CAN1/1
  Bus Creator/1 -> CAN1_msg/1
  Constant/1 -> Bus Creator/1
  Subsystem/3(board_id) -> Terminator/1

== system HANcoder_E407_TTA_Group2/HANcoder STM32 Target - E407-STM32 algorithm/TTA CAN System/TTA System/Matrix Cycle Manager/Vehicle Emulator Matrix Cycle/vehicle emulator basic cycle 1/COMP Task - Sync bc1 check/Process_Messages/Demux message CAN1 and check coherence1 ==
  CAN2_Rx_msg : Inport  OutDataTypeStr=Bus: msg_buffer_type
  expected_basic_cycle : Inport  Port=2
  Enable : EnablePort
  Bus Creator : BusCreator  Inputs=8  OutDataTypeStr=Bus: msg_buffer_type
  Bus Selector : BusSelector  OutputSignals=Buffer_1,Buffer_2,Buffer_3,Buffer_4,Buffer_5,Buffer_6,Buffer_7,Buffer_8
  Constant : Constant  Value=0  OutDataTypeStr=uint8
  Equal1 : RelationalOperator  Operator===  OutDataTypeStr=boolean  RndMeth=Simplest
  Subsystem : Subsystem
  Terminator : Terminator
  msg_count>2_DEBUG : Subsystem
  CAN2_msg_coherent : Outport  OutputWhenDisabled=reset  InitialOutput=0
  Msg_Count_CAN2 : Outport  Port=2
  CAN2_msg : Outport  Port=3  OutDataTypeStr=Bus: msg_buffer_type
  wires:
  Bus Selector/2 -> Bus Creator/2  "<Buffer_2>"
  Bus Selector/3 -> Bus Creator/3  "<Buffer_3>"
  CAN2_Rx_msg/1 -> Bus Selector/1
  Equal1/1 -> CAN2_msg_coherent/1
  expected_basic_cycle/1 -> Equal1/2
  Bus Selector/6 -> Bus Creator/6  "<Buffer_6>"
  Bus Selector/5 -> Bus Creator/5  "<Buffer_5>"
  Bus Selector/7 -> Bus Creator/7  "<Buffer_7>"
  Bus Selector/8 -> Bus Creator/8  "<Buffer_8>"
  Bus Selector/4 -> Bus Creator/4  "<Buffer_4>"
  Bus Selector/1 -> Subsystem/1(Msg_Temporal_Data)  "<Buffer_1>"
  Subsystem/1(basic_cycle) -> Equal1/1
  Subsystem/2(msg_count) -> Msg_Count_CAN2/1, msg_count>2_DEBUG/1(msg_c)
  Bus Creator/1 -> CAN2_msg/1
  Constant/1 -> Bus Creator/1
  Subsystem/3(board_id) -> Terminator/1

== system HANcoder_E407_TTA_Group2/HANcoder STM32 Target - E407-STM32 algorithm/TTA CAN System/TTA System/Matrix Cycle Manager/Vehicle Emulator Matrix Cycle/vehicle emulator basic cycle 1/COMP Task - Sync bc1 check/Process_Messages/Desync calculation ==
  note: Estimation of the Local Time when the message was sent
  note: Desync CAN2
      | expected RX - Actual RX
  note: Desync CAN1
      | expected RX - Actual RX
  TM_COMM : Inport
  New_msg_CAN1 : Inport  Port=2
  msg_count_CAN1 : Inport  Port=3
  msg_count_CAN2 : Inport  Port=4
  Enable : EnablePort
  Constant : Constant  Value=COMM_Phase1
  Constant1 : Constant  Value=COMM_Phase2
  Data Store Read : DataStoreRead  DataStoreName=Msg_Rx_Ticks_CAN1
  Data Store Read1 : DataStoreRead  DataStoreName=Msg_Rx_Ticks_CAN2
  Data Store Write1 : DataStoreWrite  Priority=23  DataStoreName=Desync_Ticks
  Minus : Sum  Priority=21  Inputs=+-
  Minus1 : Sum  Priority=20  Inputs=+-
  Multiply : Product  Priority=10
  Multiply1 : Product  Priority=12
  Saturation : Saturate  UpperLimit=max_desync  LowerLimit=min_desync
  Sum : Sum  Priority=11  Inputs=+++
  Sum1 : Sum  Priority=13  Inputs=+++
  Switch1 : Switch  Priority=22  Criteria=u2 > Threshold
  delay_estimation_1 : Constant  Value=comm_delay_estimation1
  delay_estimation_2 : Constant  Value=comm_delay_estimation2
  wires:
  TM_COMM/1 -> Sum1/2, Sum/2
  delay_estimation_1/1 -> Sum/3
  msg_count_CAN1/1 -> Multiply/2
  Switch1/1 -> Saturation/1
  Minus/1 -> Switch1/3
  Sum1/1 -> [expected_LT_CAN2]
  delay_estimation_2/1 -> Sum1/3
  Multiply1/1 -> Sum1/1
  [expected_LT_CAN1] -> Minus1/1
  [expected_LT_CAN2] -> Minus/1
  Data Store Read1/1 -> Minus/2
  Multiply/1 -> Sum/1
  Data Store Read/1 -> Minus1/2
  msg_count_CAN2/1 -> Multiply1/2
  Sum/1 -> [expected_LT_CAN1]
  Minus1/1 -> Switch1/1
  Constant/1 -> Multiply/1
  Constant1/1 -> Multiply1/1
  New_msg_CAN1/1 -> Switch1/2
  Saturation/1 -> Data Store Write1/1  "Desync_Sync_bc1_vem_s"

== system HANcoder_E407_TTA_Group2/HANcoder STM32 Target - E407-STM32 algorithm/TTA CAN System/TTA System/Matrix Cycle Manager/Vehicle Emulator Matrix Cycle/vehicle emulator basic cycle 1/COMP Task - Update LT/Local Time Update/Desync_Negative ==
  note: Local Time Update
  note: Current Local Time correction
  note: Local time correction when Desync is negative
      | In this case the Local Time "goes back in time".
      | Previous tasks will not be activated because
      | sync_processed flag is alread set.
  Current_Local_Time : Inport
  Enable : EnablePort
  Cast : DataTypeConversion  Priority=13  OutDataTypeStr=uint16
  Data Store Read : DataStoreRead  Priority=11  DataStoreName=Desync_Ticks
  Data Store Write1 : DataStoreWrite  Priority=14  DataStoreName=Local_Ticks  DataStoreElements=Local_Ticks
  Minus : Sum  Priority=12
  wires:
  Current_Local_Time/1 -> Minus/1
  Cast/1 -> Data Store Write1/1
  Minus/1 -> Cast/1
  Data Store Read/1 -> Minus/2

== system HANcoder_E407_TTA_Group2/HANcoder STM32 Target - E407-STM32 algorithm/TTA CAN System/TTA System/Matrix Cycle Manager/Controller Matrix Cycle/controller basic cycle 0/COMM Task - Sync bc 0/Transmission subtasks/Check msg transmission CAN1/TX buffer update CAN1 ==
  note: Transmission end - Set message to send through CAN 1
  note: Message Temporal Data
      |    Every message sends
      |    BasicCycle, Tx count
      |    and Verification msg
      |    as data
  note: Transmission ID
      |    Sync Msg: 1
      |    Vote Node 1: 11
      |    Vote Node 2: 12
      |    Vote Node 3: 13
  Tx_ID : Inport
  Msg_Value_Data : Inport  Port=2
  Enable : EnablePort
  Bus Selector : BusSelector  OutputSignals=signal2,signal3,signal4,signal5,signal6,signal7,signal8
  Cast : DataTypeConversion  OutDataTypeStr=uint32
  Cast1 : DataTypeConversion  OutDataTypeStr=uint8
  Cast16 : DataTypeConversion  OutDataTypeStr=uint8
  Cast4 : DataTypeConversion  OutDataTypeStr=uint8
  Data Store Read : DataStoreRead  Priority=50  DataStoreName=Tx_msg_count_CAN1
  Data Store Read1 : DataStoreRead  DataStoreName=Board_ID
  Data Store Read3 : DataStoreRead  DataStoreName=basic_cycle_count
  Data Store Write10 : DataStoreWrite  DataStoreName=Msg_Tx_CAN1  DataStoreElements=Msg_Tx_CAN1.Buffer_1#Msg_Tx_CAN1.Buffer_2#Msg_Tx_CAN1.Buffer_3#Msg_Tx_CAN1.Buffer_4#Msg_Tx_CAN1.Buffer_5#Msg_Tx_CAN1.Buffer_6#Msg_Tx_CAN1.Buffer_7#Msg_Tx_CAN1.Buffer_8
  Data Store Write8 : DataStoreWrite  DataStoreName=TxID_CAN1
  Msg_Data_Encoder : Subsystem
  wires:
  Cast/1 -> Data Store Write8/1
  Data Store Read3/1 -> Cast4/1
  Cast4/1 -> Msg_Data_Encoder/1(basic_cycle)
  Msg_Value_Data/1 -> Bus Selector/1
  Tx_ID/1 -> Cast/1
  Data Store Read/1 -> Cast1/1
  Cast16/1 -> Msg_Data_Encoder/3(board_number)
  Cast1/1 -> Msg_Data_Encoder/2(tx_counter)
  Data Store Read1/1 -> Cast16/1
  Msg_Data_Encoder/1(encoded_msg) -> Data Store Write10/1
  Bus Selector/1 -> Data Store Write10/2  "<signal2>"
  Bus Selector/2 -> Data Store Write10/3  "<signal3>"
  Bus Selector/3 -> Data Store Write10/4  "<signal4>"
  Bus Selector/4 -> Data Store Write10/5  "<signal5>"
  Bus Selector/5 -> Data Store Write10/6  "<signal6>"
  Bus Selector/6 -> Data Store Write10/7  "<signal7>"
  Bus Selector/7 -> Data Store Write10/8  "<signal8>"

== system HANcoder_E407_TTA_Group2/HANcoder STM32 Target - E407-STM32 algorithm/TTA CAN System/TTA System/Matrix Cycle Manager/Controller Matrix Cycle/controller basic cycle 0/COMM Task - Sync bc 0/Transmission subtasks/Check msg transmission CAN2/TX buffer update CAN2 ==
  note: Transmission end - Set message to send through CAN
  note: Transmission ID
      |    Sync Msg: 1
      |    Vote Node 1: 11
      |    Vote Node 2: 12
      |    Vote Node 3: 13
  note: Message Data
      |    Every message sends
      |    BasicCycle, Tx count
      |    and Verification msg
      |    as data
  Tx_ID : Inport
  Msg_Value_Data : Inport  Port=2
  Enable : EnablePort
  Bus Selector : BusSelector  OutputSignals=signal2,signal3,signal4,signal5,signal6,signal7,signal8
  Cast17 : DataTypeConversion  OutDataTypeStr=uint8
  Cast18 : DataTypeConversion  OutDataTypeStr=uint8
  Cast8 : DataTypeConversion  OutDataTypeStr=uint32
  Cast9 : DataTypeConversion  OutDataTypeStr=uint8
  Data Store Read : DataStoreRead  DataStoreName=Board_ID
  Data Store Read1 : DataStoreRead  Priority=50  DataStoreName=Tx_msg_count_CAN2
  Data Store Read6 : DataStoreRead  DataStoreName=basic_cycle_count
  Data Store Write4 : DataStoreWrite  DataStoreName=Msg_Tx_CAN2  DataStoreElements=Msg_Tx_CAN2.Buffer_1#Msg_Tx_CAN2.Buffer_2#Msg_Tx_CAN2.Buffer_3#Msg_Tx_CAN2.Buffer_4#Msg_Tx_CAN2.Buffer_5#Msg_Tx_CAN2.Buffer_6#Msg_Tx_CAN2.Buffer_7#Msg_Tx_CAN2.Buffer_8
  Data Store Write5 : DataStoreWrite  DataStoreName=TxID_CAN2
  Msg_Data_Encoder : Subsystem
  wires:
  Bus Selector/7 -> Data Store Write4/8  "<signal8>"
  Bus Selector/6 -> Data Store Write4/7  "<signal7>"
  Bus Selector/5 -> Data Store Write4/6  "<signal6>"
  Bus Selector/4 -> Data Store Write4/5  "<signal5>"
  Bus Selector/3 -> Data Store Write4/4  "<signal4>"
  Bus Selector/2 -> Data Store Write4/3  "<signal3>"
  Bus Selector/1 -> Data Store Write4/2  "<signal2>"
  Msg_Value_Data/1 -> Bus Selector/1
  Data Store Read/1 -> Cast17/1
  Cast8/1 -> Data Store Write5/1
  Cast9/1 -> Msg_Data_Encoder/2(tx_counter)
  Tx_ID/1 -> Cast8/1
  Cast17/1 -> Msg_Data_Encoder/3(verif_value)
  Data Store Read6/1 -> Cast18/1
  Msg_Data_Encoder/1(encoded_msg) -> Data Store Write4/1
  Data Store Read1/1 -> Cast9/1
  Cast18/1 -> Msg_Data_Encoder/1(basic_cycle)

== system HANcoder_E407_TTA_Group2/HANcoder STM32 Target - E407-STM32 algorithm/TTA CAN System/TTA System/Matrix Cycle Manager/Controller Matrix Cycle/controller basic cycle 0/COMM Task - Vote1/Transmission subtasks/Check msg transmission CAN1/TX buffer update CAN1 ==
  note: Transmission end - Set message to send through CAN 1
  note: Message Temporal Data
      |    Every message sends
      |    BasicCycle, Tx count
      |    and Verification msg
      |    as data
  note: Transmission ID
      |    Sync Msg: 1
      |    Vote Node 1: 11
      |    Vote Node 2: 12
      |    Vote Node 3: 13
  Tx_ID : Inport
  Msg_Value_Data : Inport  Port=2
  Enable : EnablePort
  Bus Selector : BusSelector  OutputSignals=signal2,signal3,signal4,signal5,signal6,signal7,signal8
  Cast : DataTypeConversion  OutDataTypeStr=uint32
  Cast1 : DataTypeConversion  OutDataTypeStr=uint8
  Cast16 : DataTypeConversion  OutDataTypeStr=uint8
  Cast4 : DataTypeConversion  OutDataTypeStr=uint8
  Data Store Read : DataStoreRead  Priority=50  DataStoreName=Tx_msg_count_CAN1
  Data Store Read1 : DataStoreRead  DataStoreName=Board_ID
  Data Store Read3 : DataStoreRead  DataStoreName=basic_cycle_count
  Data Store Write10 : DataStoreWrite  DataStoreName=Msg_Tx_CAN1  DataStoreElements=Msg_Tx_CAN1.Buffer_1#Msg_Tx_CAN1.Buffer_2#Msg_Tx_CAN1.Buffer_3#Msg_Tx_CAN1.Buffer_4#Msg_Tx_CAN1.Buffer_5#Msg_Tx_CAN1.Buffer_6#Msg_Tx_CAN1.Buffer_7#Msg_Tx_CAN1.Buffer_8
  Data Store Write8 : DataStoreWrite  DataStoreName=TxID_CAN1
  Msg_Data_Encoder : Subsystem
  wires:
  Cast/1 -> Data Store Write8/1
  Data Store Read3/1 -> Cast4/1
  Cast4/1 -> Msg_Data_Encoder/1(basic_cycle)
  Msg_Value_Data/1 -> Bus Selector/1
  Tx_ID/1 -> Cast/1
  Data Store Read/1 -> Cast1/1
  Cast16/1 -> Msg_Data_Encoder/3(board_number)
  Cast1/1 -> Msg_Data_Encoder/2(tx_counter)
  Data Store Read1/1 -> Cast16/1
  Msg_Data_Encoder/1(encoded_msg) -> Data Store Write10/1
  Bus Selector/1 -> Data Store Write10/2  "<signal2>"
  Bus Selector/2 -> Data Store Write10/3  "<signal3>"
  Bus Selector/3 -> Data Store Write10/4  "<signal4>"
  Bus Selector/4 -> Data Store Write10/5  "<signal5>"
  Bus Selector/5 -> Data Store Write10/6  "<signal6>"
  Bus Selector/6 -> Data Store Write10/7  "<signal7>"
  Bus Selector/7 -> Data Store Write10/8  "<signal8>"

== system HANcoder_E407_TTA_Group2/HANcoder STM32 Target - E407-STM32 algorithm/TTA CAN System/TTA System/Matrix Cycle Manager/Controller Matrix Cycle/controller basic cycle 0/COMM Task - Vote1/Transmission subtasks/Check msg transmission CAN2/TX buffer update CAN2 ==
  note: Transmission end - Set message to send through CAN
  note: Transmission ID
      |    Sync Msg: 1
      |    Vote Node 1: 11
      |    Vote Node 2: 12
      |    Vote Node 3: 13
  note: Message Data
      |    Every message sends
      |    BasicCycle, Tx count
      |    and Verification msg
      |    as data
  Tx_ID : Inport
  Msg_Value_Data : Inport  Port=2
  Enable : EnablePort
  Bus Selector : BusSelector  OutputSignals=signal2,signal3,signal4,signal5,signal6,signal7,signal8
  Cast17 : DataTypeConversion  OutDataTypeStr=uint8
  Cast18 : DataTypeConversion  OutDataTypeStr=uint8
  Cast8 : DataTypeConversion  OutDataTypeStr=uint32
  Cast9 : DataTypeConversion  OutDataTypeStr=uint8
  Data Store Read : DataStoreRead  DataStoreName=Board_ID
  Data Store Read1 : DataStoreRead  Priority=50  DataStoreName=Tx_msg_count_CAN2
  Data Store Read6 : DataStoreRead  DataStoreName=basic_cycle_count
  Data Store Write4 : DataStoreWrite  DataStoreName=Msg_Tx_CAN2  DataStoreElements=Msg_Tx_CAN2.Buffer_1#Msg_Tx_CAN2.Buffer_2#Msg_Tx_CAN2.Buffer_3#Msg_Tx_CAN2.Buffer_4#Msg_Tx_CAN2.Buffer_5#Msg_Tx_CAN2.Buffer_6#Msg_Tx_CAN2.Buffer_7#Msg_Tx_CAN2.Buffer_8
  Data Store Write5 : DataStoreWrite  DataStoreName=TxID_CAN2
  Msg_Data_Encoder : Subsystem
  wires:
  Bus Selector/7 -> Data Store Write4/8  "<signal8>"
  Bus Selector/6 -> Data Store Write4/7  "<signal7>"
  Bus Selector/5 -> Data Store Write4/6  "<signal6>"
  Bus Selector/4 -> Data Store Write4/5  "<signal5>"
  Bus Selector/3 -> Data Store Write4/4  "<signal4>"
  Bus Selector/2 -> Data Store Write4/3  "<signal3>"
  Bus Selector/1 -> Data Store Write4/2  "<signal2>"
  Msg_Value_Data/1 -> Bus Selector/1
  Data Store Read/1 -> Cast17/1
  Cast8/1 -> Data Store Write5/1
  Cast9/1 -> Msg_Data_Encoder/2(tx_counter)
  Tx_ID/1 -> Cast8/1
  Cast17/1 -> Msg_Data_Encoder/3(verif_value)
  Data Store Read6/1 -> Cast18/1
  Msg_Data_Encoder/1(encoded_msg) -> Data Store Write4/1
  Data Store Read1/1 -> Cast9/1
  Cast18/1 -> Msg_Data_Encoder/1(basic_cycle)

== system HANcoder_E407_TTA_Group2/HANcoder STM32 Target - E407-STM32 algorithm/TTA CAN System/TTA System/Matrix Cycle Manager/Controller Matrix Cycle/controller basic cycle 0/COMM Task - Vote2/Transmission subtasks/Check msg transmission CAN1/TX buffer update CAN1 ==
  note: Transmission end - Set message to send through CAN 1
  note: Message Temporal Data
      |    Every message sends
      |    BasicCycle, Tx count
      |    and Verification msg
      |    as data
  note: Transmission ID
      |    Sync Msg: 1
      |    Vote Node 1: 11
      |    Vote Node 2: 12
      |    Vote Node 3: 13
  Tx_ID : Inport
  Msg_Value_Data : Inport  Port=2
  Enable : EnablePort
  Bus Selector : BusSelector  OutputSignals=signal2,signal3,signal4,signal5,signal6,signal7,signal8
  Cast : DataTypeConversion  OutDataTypeStr=uint32
  Cast1 : DataTypeConversion  OutDataTypeStr=uint8
  Cast16 : DataTypeConversion  OutDataTypeStr=uint8
  Cast4 : DataTypeConversion  OutDataTypeStr=uint8
  Data Store Read : DataStoreRead  Priority=50  DataStoreName=Tx_msg_count_CAN1
  Data Store Read1 : DataStoreRead  DataStoreName=Board_ID
  Data Store Read3 : DataStoreRead  DataStoreName=basic_cycle_count
  Data Store Write10 : DataStoreWrite  DataStoreName=Msg_Tx_CAN1  DataStoreElements=Msg_Tx_CAN1.Buffer_1#Msg_Tx_CAN1.Buffer_2#Msg_Tx_CAN1.Buffer_3#Msg_Tx_CAN1.Buffer_4#Msg_Tx_CAN1.Buffer_5#Msg_Tx_CAN1.Buffer_6#Msg_Tx_CAN1.Buffer_7#Msg_Tx_CAN1.Buffer_8
  Data Store Write8 : DataStoreWrite  DataStoreName=TxID_CAN1
  Msg_Data_Encoder : Subsystem
  wires:
  Cast/1 -> Data Store Write8/1
  Data Store Read3/1 -> Cast4/1
  Cast4/1 -> Msg_Data_Encoder/1(basic_cycle)
  Msg_Value_Data/1 -> Bus Selector/1
  Tx_ID/1 -> Cast/1
  Data Store Read/1 -> Cast1/1
  Cast16/1 -> Msg_Data_Encoder/3(board_number)
  Cast1/1 -> Msg_Data_Encoder/2(tx_counter)
  Data Store Read1/1 -> Cast16/1
  Msg_Data_Encoder/1(encoded_msg) -> Data Store Write10/1
  Bus Selector/1 -> Data Store Write10/2  "<signal2>"
  Bus Selector/2 -> Data Store Write10/3  "<signal3>"
  Bus Selector/3 -> Data Store Write10/4  "<signal4>"
  Bus Selector/4 -> Data Store Write10/5  "<signal5>"
  Bus Selector/5 -> Data Store Write10/6  "<signal6>"
  Bus Selector/6 -> Data Store Write10/7  "<signal7>"
  Bus Selector/7 -> Data Store Write10/8  "<signal8>"

== system HANcoder_E407_TTA_Group2/HANcoder STM32 Target - E407-STM32 algorithm/TTA CAN System/TTA System/Matrix Cycle Manager/Controller Matrix Cycle/controller basic cycle 0/COMM Task - Vote2/Transmission subtasks/Check msg transmission CAN2/TX buffer update CAN2 ==
  note: Transmission end - Set message to send through CAN
  note: Transmission ID
      |    Sync Msg: 1
      |    Vote Node 1: 11
      |    Vote Node 2: 12
      |    Vote Node 3: 13
  note: Message Data
      |    Every message sends
      |    BasicCycle, Tx count
      |    and Verification msg
      |    as data
  Tx_ID : Inport
  Msg_Value_Data : Inport  Port=2
  Enable : EnablePort
  Bus Selector : BusSelector  OutputSignals=signal2,signal3,signal4,signal5,signal6,signal7,signal8
  Cast17 : DataTypeConversion  OutDataTypeStr=uint8
  Cast18 : DataTypeConversion  OutDataTypeStr=uint8
  Cast8 : DataTypeConversion  OutDataTypeStr=uint32
  Cast9 : DataTypeConversion  OutDataTypeStr=uint8
  Data Store Read : DataStoreRead  DataStoreName=Board_ID
  Data Store Read1 : DataStoreRead  Priority=50  DataStoreName=Tx_msg_count_CAN2
  Data Store Read6 : DataStoreRead  DataStoreName=basic_cycle_count
  Data Store Write4 : DataStoreWrite  DataStoreName=Msg_Tx_CAN2  DataStoreElements=Msg_Tx_CAN2.Buffer_1#Msg_Tx_CAN2.Buffer_2#Msg_Tx_CAN2.Buffer_3#Msg_Tx_CAN2.Buffer_4#Msg_Tx_CAN2.Buffer_5#Msg_Tx_CAN2.Buffer_6#Msg_Tx_CAN2.Buffer_7#Msg_Tx_CAN2.Buffer_8
  Data Store Write5 : DataStoreWrite  DataStoreName=TxID_CAN2
  Msg_Data_Encoder : Subsystem
  wires:
  Bus Selector/7 -> Data Store Write4/8  "<signal8>"
  Bus Selector/6 -> Data Store Write4/7  "<signal7>"
  Bus Selector/5 -> Data Store Write4/6  "<signal6>"
  Bus Selector/4 -> Data Store Write4/5  "<signal5>"
  Bus Selector/3 -> Data Store Write4/4  "<signal4>"
  Bus Selector/2 -> Data Store Write4/3  "<signal3>"
  Bus Selector/1 -> Data Store Write4/2  "<signal2>"
  Msg_Value_Data/1 -> Bus Selector/1
  Data Store Read/1 -> Cast17/1
  Cast8/1 -> Data Store Write5/1
  Cast9/1 -> Msg_Data_Encoder/2(tx_counter)
  Tx_ID/1 -> Cast8/1
  Cast17/1 -> Msg_Data_Encoder/3(verif_value)
  Data Store Read6/1 -> Cast18/1
  Msg_Data_Encoder/1(encoded_msg) -> Data Store Write4/1
  Data Store Read1/1 -> Cast9/1
  Cast18/1 -> Msg_Data_Encoder/1(basic_cycle)
